simulink model "Electromecanico_sim"  (R2023b)
settings: Solver=ode45  StartTime=0.0  StopTime=10.0  RelTol=1e-3
values from neighbouring files (symbols this model uses):
  b = 0.0012    [Condiciones.mat]    (also in electromecanico.m)
  J = 0.001    [Condiciones.mat]    (also in electromecanico.m)
  Ke = 0.01    [Condiciones.mat]    (also in electromecanico.m)
  Kt = 0.01    [Condiciones.mat]    (also in electromecanico.m)
  La = 0.023    [Condiciones.mat]    (also in electromecanico.m)
  Ra = 2    [Condiciones.mat]    (also in electromecanico.m)
  T = 0    [Condiciones.mat]    (also in electromecanico.m)
settings Model: Creator=andre  LastModifiedBy=andre

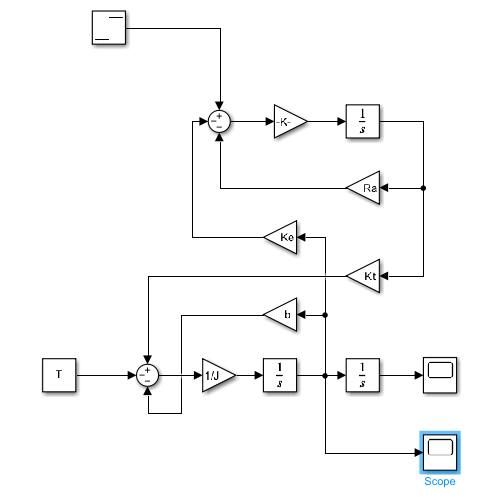
[thumbnail: Simulink's stored preview of the top-level diagram]
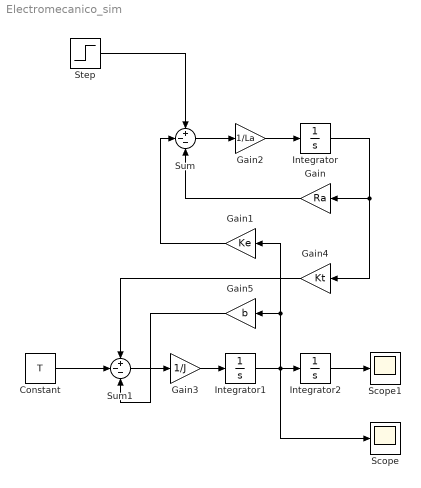
== system Electromecanico_sim ==
  Constant : Constant  Value=T
  Gain : Gain  Gain=Ra
  Gain1 : Gain  Gain=Ke
  Gain2 : Gain  Gain=1/La
  Gain3 : Gain  Gain=1/J
  Gain4 : Gain  Gain=Kt
  Gain5 : Gain  Gain=b
  Integrator : Integrator
  Integrator1 : Integrator
  Integrator2 : Integrator
  Scope : Scope
  Scope1 : Scope
  Step : Step  Time=0  After=5  SampleTime=0
  Sum : Sum  Inputs=+--
  Sum1 : Sum  Inputs=+--
  wires:
  Integrator1/1 -> Gain1/1, Gain5/1, Scope/1, Integrator2/1
  Step/1 -> Sum/1
  Integrator/1 -> Gain/1, Gain4/1
  Gain/1 -> Sum/3
  Gain1/1 -> Sum/2
  Sum/1 -> Gain2/1
  Gain2/1 -> Integrator/1
  Gain3/1 -> Integrator1/1
  Sum1/1 -> Gain3/1
  Gain4/1 -> Sum1/1
  Constant/1 -> Sum1/2
  Gain5/1 -> Sum1/3
  Integrator2/1 -> Scope1/1
